simulink model "test_ABCD"  (R2020b)
settings: Solver=FixedStepAuto  StartTime=0.0  StopTime=10.0  RelTol=1e-3
undefined symbols (not defined in the file or in its folder): A_matrix, B_matrix, C_matrix, D_matrix
settings Model: Creator=Alexi  LastModifiedBy=Alexi

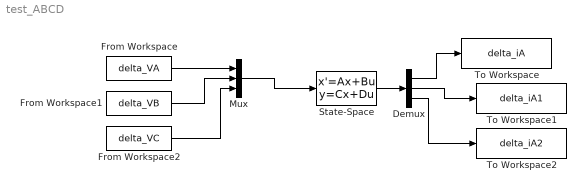
== system test_ABCD ==
  Demux : Demux  Outputs=3
  From Workspace : FromWorkspace  VariableName=delta_VA
  From Workspace1 : FromWorkspace  VariableName=delta_VB
  From Workspace2 : FromWorkspace  VariableName=delta_VC
  Mux : Mux  Inputs=3
  State-Space : StateSpace  A=A_matrix  B=B_matrix  C=C_matrix  D=D_matrix  InitialCondition=0  ContinuousStateAttributes={'delta_iA', 'delta_iB', 'delta_iC'}
  To Workspace : ToWorkspace  VariableName=delta_iA  SaveFormat=Timeseries  SampleTime=-1
  To Workspace1 : ToWorkspace  VariableName=delta_iA1  SaveFormat=Timeseries  SampleTime=-1
  To Workspace2 : ToWorkspace  VariableName=delta_iA2  SaveFormat=Timeseries  SampleTime=-1
  wires:
  From Workspace/1 -> Mux/1
  From Workspace1/1 -> Mux/2
  From Workspace2/1 -> Mux/3
  Mux/1 -> State-Space/1
  State-Space/1 -> Demux/1
  Demux/1 -> To Workspace/1
  Demux/2 -> To Workspace1/1
  Demux/3 -> To Workspace2/1
